simulink model "rtwdemo_minmax"  (Simulink 7.6)
settings: Solver=FixedStepDiscrete  StartTime=0.0  StopTime=10.0  FixedStep=0.2  RelTol=1e-3
PreLoadFcn:
  | k=Simulink.Parameter; k.Value=15; k.RTWInfo.StorageClass='ExportedGlobal';
libraries: rtwdemowidgets x2
Description:
  | Code Optimizations Based On Specified Mininimum and Maximum Values
settings Model: Creator=The MathWorks Inc.
settings DataIOCC: SaveOutput=off  SaveTime=off
settings OptimizationCC: InlineParams=on  UseIntDivNetSlope=on  InlineInvariantSignals=on  EnhancedBackFolding=on  BooleansAsBitfields=on  PassReuseOutputArgsAs=Individual arguments  StateBitsets=on  DataBitsets=on  UseTempVars=on  ZeroExternalMemoryAtStartup=off  ZeroInternalMemoryAtStartup=off  NoFixptDivByZeroProtection=on  EfficientFloat2IntCast=on  OptimizeModelRefInitCode=on  LifeSpan=1
settings DebuggingCC: UnderspecifiedInitializationDetection=Simplified  MergeDetectMultiDrivingBlocksExec=error  FcnCallInpInsideContextMsg=Enable All  UniqueDataStoreMsg=error  AssertControl=DisableAll  StrictBusMsg=ErrorOnBusTreatedAsVector
settings HardwareCC: ProdIntDivRoundTo=Zero  ProdEndianess=LittleEndian  ProdHWDeviceType=Generic->32-bit Embedded Processor
settings RTWCC: SystemTargetFile=ert.tlc  TemplateMakefile=ert_default_tmf  Description=Real-Time Workshop Embedded Coder  GenerateReport=on  RTWVerbose=off  ProcessScript=ert_make_rtw_hook  IncludeHyperlinkInReport=on  LaunchReport=on  GenerateTraceInfo=on  GenerateTraceReport=on  GenerateTraceReportSl=on  GenerateTraceReportSf=on  GenerateTraceReportEml=on
settings CodeAppCC: ForceParamTrailComments=on  IgnoreCustomStorageClasses=off  IgnoreTestpoints=on  SimulinkDataObjDesc=on  CustomSymbolStrGlobalVar=rt$N$M  CustomSymbolStrType=$N$M  CustomSymbolStrFcn=$N$M$F  CustomSymbolStrMacro=$N$M  InsertBlockDesc=on
settings ERTTargetCC: MultiwordLength=2048  GenerateSampleERTMain=on  IncludeMdlTerminateFcn=off  CombineSignalStateStructs=on  SupportNonFinite=off  SupportComplex=off  ParenthesesLevel=Maximum  ERTCustomFileTemplate=example_file_process.tlc  ERTFilePackagingFormat=CompactWithDataFile  ConvertIfToSwitch=off

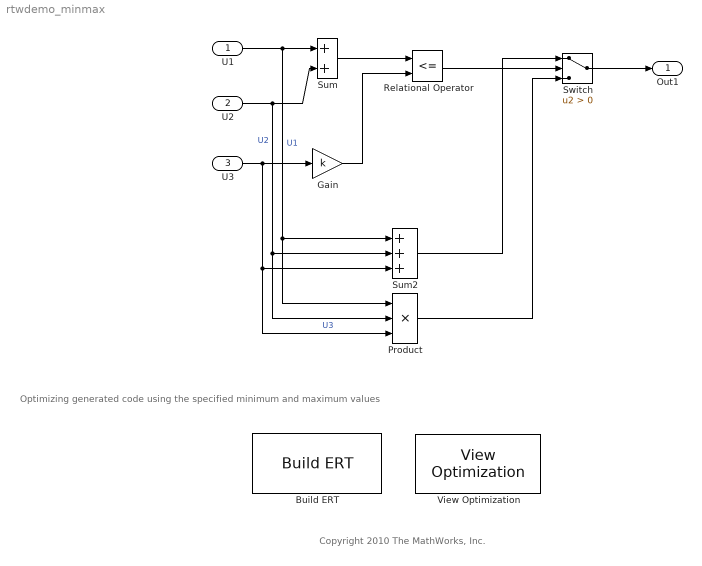
== system rtwdemo_minmax ==
  note: Copyright 2010 The MathWorks, Inc.
  note: Optimizing generated code using the specified minimum and maximum values
  U1 : Inport  OutMin=50  OutMax=100  OutDataTypeStr=int8
      settings: AttributesFormatString=Min=%<OutMin>\nMax=%<OutMax>
  U2 : Inport  Port=2  OutMin=0  OutDataTypeStr=int8
      settings: AttributesFormatString=Min=%<OutMin>
  U3 : Inport  Port=3  OutMax=2  OutDataTypeStr=int8
      settings: AttributesFormatString=Max=%<OutMax>
  Build ERT : rtwdemowidgets/Build ERT  SystemSampleTime=-1  attrib_overrides={}
  Gain : Gain  Gain=k  ParamMin=10  ParamMax=20  ParamDataTypeStr=int8  OutDataTypeStr=int32
      settings: AttributesFormatString=Param Min=%<ParamMin>\nParam Max=%<ParamMax>
  Product : Product  Inputs=3  OutDataTypeStr=int32  RndMeth=Zero
  Relational Operator : RelationalOperator  Operator=<=  OutDataTypeStr=boolean
  Sum : Sum  OutDataTypeStr=int32
      settings: AttributesFormatString=%<Name>
  Sum2 : Sum  Inputs=+++  OutDataTypeStr=int32
      settings: AttributesFormatString=%<Name>
  Switch : Switch  Criteria=u2 > Threshold
  View Optimization : rtwdemowidgets/View Optimization  SystemSampleTime=-1
  Out1 : Outport
  wires:
  U1/1 -> Sum/1, Product/1, Sum2/1  "U1"
  U2/1 -> Sum/2, Product/2, Sum2/2  "U2"
  U3/1 -> Product/3, Sum2/3, Gain/1  "U3"
  Sum/1 -> Relational Operator/1
  Gain/1 -> Relational Operator/2
  Relational Operator/1 -> Switch/2
  Switch/1 -> Out1/1
  Sum2/1 -> Switch/1
  Product/1 -> Switch/3
